simulink model "DalinovRegulatorNaDrugiNacin"  (R2013b)
settings: Solver=ode45  StartTime=0.0  StopTime=10.0  RelTol=1e-3
settings Model: Creator=Darko  LastModifiedBy=Darko

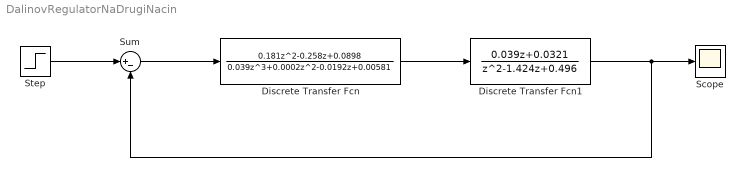
== system DalinovRegulatorNaDrugiNacin ==
  Discrete Transfer Fcn : DiscreteTransferFcn  Numerator=[0.181 -0.258 0.0898]  Denominator=[0.039 0.0002 -0.0192 0.00581]  SampleTime=0.1
  Discrete Transfer Fcn1 : DiscreteTransferFcn  Numerator=[0.039 0.0321]  Denominator=[1 -1.424 0.496]  SampleTime=0.1
  Scope : Scope
  Step : Step  Time=0  SampleTime=0.01
  Sum : Sum  Inputs=|+-
  wires:
  Step/1 -> Sum/1
  Sum/1 -> Discrete Transfer Fcn/1
  Discrete Transfer Fcn/1 -> Discrete Transfer Fcn1/1
  Discrete Transfer Fcn1/1 -> Sum/2, Scope/1
